simulink model "write16bits"  (R2015b)
settings: Solver=ode45  StartTime=0.0  StopTime=10.0  RelTol=1e-3
undefined symbols (not defined in the file or in its folder): A7, A8, B7, B8, C5, F15, L3, M14, M3, N15, N3, P3, PC11, PC12, PC13, PC14, PC15, PD0, PD1, PD10, PD2, PD3, PD4, PD5, PD6, PD7, PD8, PD9, R4, T15
libraries: simulink x16, rappid_564xl_ec_toolbox x16
settings Model: Creator=Riley  LastModifiedBy=jfr
settings DataIOCC: SaveFormat=Array
settings OptimizationCC: ExpressionDepthLimit=2147483647
settings DebuggingCC: UnderspecifiedInitializationDetection=Classic  MergeDetectMultiDrivingBlocksExec=none  SolverPrmCheckMsg=warning  FcnCallInpInsideContextMsg=EnableAllAsWarning  StateNameClashWarn=warning
settings HardwareCC: ProdBitPerPointer=32  ProdLargestAtomicFloat=None  ProdIntDivRoundTo=Undefined  ProdEndianess=Unspecified  ProdWordSize=32  ProdHWDeviceType=32-bit Generic
settings GRTTargetCC: GeneratePreprocessorConditionals=Disable all  CombineOutputUpdateFcns=off  GRTInterface=on
settings ConfigComp: CovModelRefEnable=Off

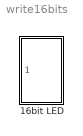
== system write16bits ==
  16bit LED : Subsystem

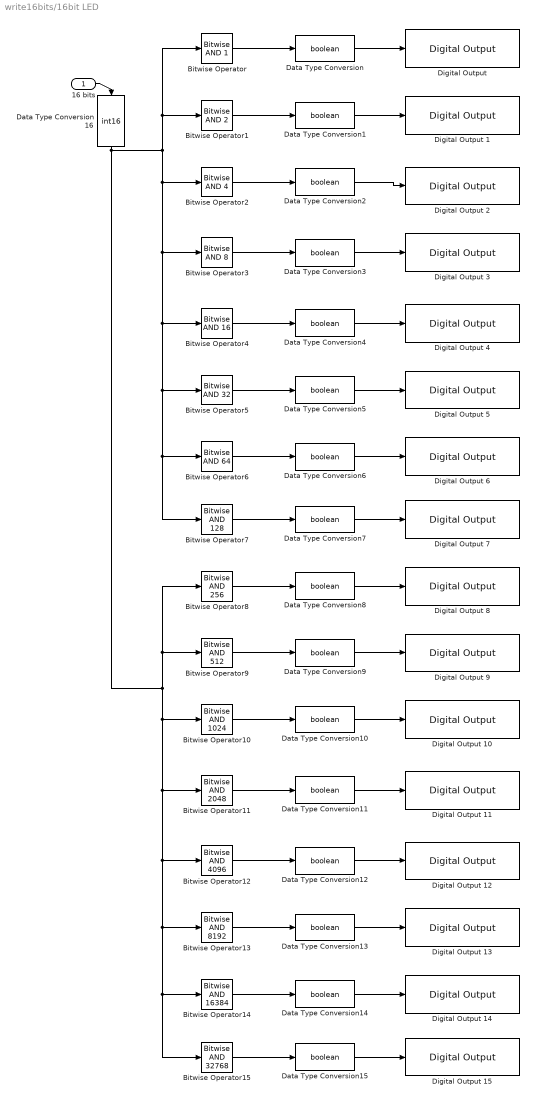
== system write16bits/16bit LED ==
  16 bits : Inport
  Bitwise Operator : simulink/Logic and Bit Operations/Bitwise Operator  logicop=AND  UseBitMask=on  BitMask=1  BitMaskRealWorld=Stored Integer
  Bitwise Operator1 : simulink/Logic and Bit Operations/Bitwise Operator  logicop=AND  UseBitMask=on  BitMask=2  BitMaskRealWorld=Stored Integer
  Bitwise Operator10 : simulink/Logic and Bit Operations/Bitwise Operator  logicop=AND  UseBitMask=on  BitMask=1024  BitMaskRealWorld=Stored Integer
  Bitwise Operator11 : simulink/Logic and Bit Operations/Bitwise Operator  logicop=AND  UseBitMask=on  BitMask=2048  BitMaskRealWorld=Stored Integer
  Bitwise Operator12 : simulink/Logic and Bit Operations/Bitwise Operator  logicop=AND  UseBitMask=on  BitMask=4096  BitMaskRealWorld=Stored Integer
  Bitwise Operator13 : simulink/Logic and Bit Operations/Bitwise Operator  logicop=AND  UseBitMask=on  BitMask=8192  BitMaskRealWorld=Stored Integer
  Bitwise Operator14 : simulink/Logic and Bit Operations/Bitwise Operator  logicop=AND  UseBitMask=on  BitMask=16384  BitMaskRealWorld=Stored Integer
  Bitwise Operator15 : simulink/Logic and Bit Operations/Bitwise Operator  logicop=AND  UseBitMask=on  BitMask=32768  BitMaskRealWorld=Stored Integer
  Bitwise Operator2 : simulink/Logic and Bit Operations/Bitwise Operator  logicop=AND  UseBitMask=on  BitMask=4  BitMaskRealWorld=Stored Integer
  Bitwise Operator3 : simulink/Logic and Bit Operations/Bitwise Operator  logicop=AND  UseBitMask=on  BitMask=8  BitMaskRealWorld=Stored Integer
  Bitwise Operator4 : simulink/Logic and Bit Operations/Bitwise Operator  logicop=AND  UseBitMask=on  BitMask=16  BitMaskRealWorld=Stored Integer
  Bitwise Operator5 : simulink/Logic and Bit Operations/Bitwise Operator  logicop=AND  UseBitMask=on  BitMask=32  BitMaskRealWorld=Stored Integer
  Bitwise Operator6 : simulink/Logic and Bit Operations/Bitwise Operator  logicop=AND  UseBitMask=on  BitMask=64  BitMaskRealWorld=Stored Integer
  Bitwise Operator7 : simulink/Logic and Bit Operations/Bitwise Operator  logicop=AND  UseBitMask=on  BitMask=128  BitMaskRealWorld=Stored Integer
  Bitwise Operator8 : simulink/Logic and Bit Operations/Bitwise Operator  logicop=AND  UseBitMask=on  BitMask=256  BitMaskRealWorld=Stored Integer
  Bitwise Operator9 : simulink/Logic and Bit Operations/Bitwise Operator  logicop=AND  UseBitMask=on  BitMask=512  BitMaskRealWorld=Stored Integer
  Data Type Conversion{,1..15} (16 alike) : DataTypeConversion  OutDataTypeStr=boolean
  Data Type Conversion16 : DataTypeConversion  OutDataTypeStr=int16
  "Digital Output " : rappid_564xl_ec_toolbox/MPC564xL/General Purpose Blocks/Digital Output   gpio_outputs="43  : PC11 : [ 80 ] : [ M14 ]"  pinNum=[ 80 ]  pcrNum=43
  Digital Output 1 : rappid_564xl_ec_toolbox/MPC564xL/General Purpose Blocks/Digital Output   gpio_outputs="44  : PC12 : [ 82 ] : [ N15 ]"  pinNum=[ 82 ]  pcrNum=44
  Digital Output 10 : rappid_564xl_ec_toolbox/MPC564xL/General Purpose Blocks/Digital Output   gpio_outputs="53  : PD5  : [ 33 ] : [ N3 ]"  pinNum=[ 33 ]  pcrNum=53
  Digital Output 11 : rappid_564xl_ec_toolbox/MPC564xL/General Purpose Blocks/Digital Output   gpio_outputs="54  : PD6  : [ 34 ] : [ P3 ]"  pinNum=[ 34 ]  pcrNum=54
  Digital Output 12 : rappid_564xl_ec_toolbox/MPC564xL/General Purpose Blocks/Digital Output   gpio_outputs="55  : PD7  : [ 37 ] : [ R4 ]"  pinNum=[ 37 ]  pcrNum=55
  Digital Output 13 : rappid_564xl_ec_toolbox/MPC564xL/General Purpose Blocks/Digital Output   gpio_outputs="56  : PD8  : [ 32 ] : [ M3 ]"  pinNum=[ 32 ]  pcrNum=56
  Digital Output 14 : rappid_564xl_ec_toolbox/MPC564xL/General Purpose Blocks/Digital Output   gpio_outputs="57  : PD9  : [ 26 ] : [ L3 ]"  pinNum=[ 26 ]  pcrNum=57
  Digital Output 15 : rappid_564xl_ec_toolbox/MPC564xL/General Purpose Blocks/Digital Output   gpio_outputs="58  : PD10 : [ 76 ] : [ T15 ]"  pinNum=[ 76 ]  pcrNum=58
  Digital Output 2 : rappid_564xl_ec_toolbox/MPC564xL/General Purpose Blocks/Digital Output   gpio_outputs="45  : PC13 : [ 101 ] : [ F15 ]"  pinNum=[ 101 ]  pcrNum=45
  Digital Output 3 : rappid_564xl_ec_toolbox/MPC564xL/General Purpose Blocks/Digital Output   gpio_outputs="46  : PC14 : [ 103 ] : [ E15 ]"  pinNum=[ 103 ]  pcrNum=46
  Digital Output 4 : rappid_564xl_ec_toolbox/MPC564xL/General Purpose Blocks/Digital Output   gpio_outputs="47  : PC15 : [ 124 ] : [ A8 ]"  pinNum=[ 124 ]  pcrNum=47
  Digital Output 5 : rappid_564xl_ec_toolbox/MPC564xL/General Purpose Blocks/Digital Output   gpio_outputs="48  : PD0  : [ 125 ] : [ B8 ]"  pinNum=[ 125 ]  pcrNum=48
  Digital Output 6 : rappid_564xl_ec_toolbox/MPC564xL/General Purpose Blocks/Digital Output   gpio_outputs="49  : PD1  : [ 3 ] : [ E3 ]"  pinNum=[ 3 ]  pcrNum=49
  Digital Output 7 : rappid_564xl_ec_toolbox/MPC564xL/General Purpose Blocks/Digital Output   gpio_outputs="50  : PD2  : [ 140 ] : [ C5 ]"  pinNum=[ 140 ]  pcrNum=50
  Digital Output 8 : rappid_564xl_ec_toolbox/MPC564xL/General Purpose Blocks/Digital Output   gpio_outputs="51  : PD3  : [ 128 ] : [ A7 ]"  pinNum=[ 128 ]  pcrNum=51
  Digital Output 9 : rappid_564xl_ec_toolbox/MPC564xL/General Purpose Blocks/Digital Output   gpio_outputs="52  : PD4  : [ 129 ] : [ B7 ]"  pinNum=[ 129 ]  pcrNum=52
  wires:
  Data Type Conversion16/1 -> Bitwise Operator10/1, Bitwise Operator11/1, Bitwise Operator12/1, Bitwise Operator13/1, Bitwise Operator14/1, Bitwise Operator15/1, Bitwise Operator9/1, Bitwise Operator8/1, Bitwise Operator/1, Bitwise Operator1/1, Bitwise Operator7/1, Bitwise Operator6/1, Bitwise Operator5/1, Bitwise Operator4/1, Bitwise Operator3/1, Bitwise Operator2/1
  Bitwise Operator15/1 -> Data Type Conversion15/1
  Data Type Conversion15/1 -> Digital Output 15/1
  Bitwise Operator14/1 -> Data Type Conversion14/1
  Data Type Conversion14/1 -> Digital Output 14/1
  Bitwise Operator13/1 -> Data Type Conversion13/1
  Data Type Conversion13/1 -> Digital Output 13/1
  Bitwise Operator8/1 -> Data Type Conversion8/1
  Bitwise Operator9/1 -> Data Type Conversion9/1
  Bitwise Operator10/1 -> Data Type Conversion10/1
  Bitwise Operator11/1 -> Data Type Conversion11/1
  Bitwise Operator12/1 -> Data Type Conversion12/1
  Data Type Conversion8/1 -> Digital Output 8/1
  Data Type Conversion9/1 -> Digital Output 9/1
  Data Type Conversion10/1 -> Digital Output 10/1
  Data Type Conversion11/1 -> Digital Output 11/1
  Data Type Conversion12/1 -> Digital Output 12/1
  Bitwise Operator7/1 -> Data Type Conversion7/1
  Data Type Conversion7/1 -> Digital Output 7/1
  Bitwise Operator6/1 -> Data Type Conversion6/1
  Data Type Conversion6/1 -> Digital Output 6/1
  Bitwise Operator5/1 -> Data Type Conversion5/1
  Data Type Conversion5/1 -> Digital Output 5/1
  Bitwise Operator/1 -> Data Type Conversion/1
  Bitwise Operator1/1 -> Data Type Conversion1/1
  Bitwise Operator2/1 -> Data Type Conversion2/1
  Bitwise Operator3/1 -> Data Type Conversion3/1
  Bitwise Operator4/1 -> Data Type Conversion4/1
  16 bits/1 -> Data Type Conversion16/1
  Data Type Conversion/1 -> "Digital Output "/1
  Data Type Conversion1/1 -> Digital Output 1/1
  Data Type Conversion2/1 -> Digital Output 2/1
  Data Type Conversion3/1 -> Digital Output 3/1
  Data Type Conversion4/1 -> Digital Output 4/1
